simulink model "puma_pbvs"  (R2016a)
settings: Solver=ode45  StartTime=0.0  StopTime=20.0  RelTol=1e-3
InitFcn:
  | mdl_puma560
  | camera = CentralCamera('default');
  | P = mkgrid(2, 0.5, troty(pi/2)*transl(0,0,2.5));
  | q0 = [0 pi/4 pi 0 pi/4 -pi/4]';
undefined symbols (not defined in the file or in its folder): get_T_c_to_cdes
libraries: roblocks x8
settings Model: ExtModeTrigMode=oneshot  ExtModeArmWhenConnect=off  Creator=pic  LastModifiedBy=magiccjae
settings DataIOCC: SaveFormat=StructureWithTime  SignalLoggingSaveFormat=ModelDataLogs  ReturnWorkspaceOutputs=on
settings OptimizationCC: BlockReduction=off  BooleanDataType=off  ExpressionDepthLimit=2147483647  InitFltsAndDblsToZero=on
settings DebuggingCC: SaveWithParameterizedLinksMsg=none  UnderspecifiedInitializationDetection=Classic  MergeDetectMultiDrivingBlocksExec=none  SignalResolutionControl=TryResolveAllWithWarning  MultiTaskDSMMsg=warning  MultiTaskCondExecSysMsg=none  FcnCallInpInsideContextMsg=UseLocalSettings  StateNameClashWarn=warning
settings HardwareCC: ProdBitPerPointer=32  ProdLargestAtomicFloat=None  ProdIntDivRoundTo=Undefined  ProdEndianess=Unspecified  ProdWordSize=32  ProdHWDeviceType=32-bit Generic  TargetUnknown=on
settings ModelReferenceCC: PropagateSignalLabelsOutOfModel=off
settings GRTTargetCC: ModelReferenceCompliant=off  CompOptLevelCompliant=off  CombineOutputUpdateFcns=off  MatFileLogging=off  GRTInterface=on
settings ConfigComp: CovModelRefEnable=Off  CovSFcnEnable=off

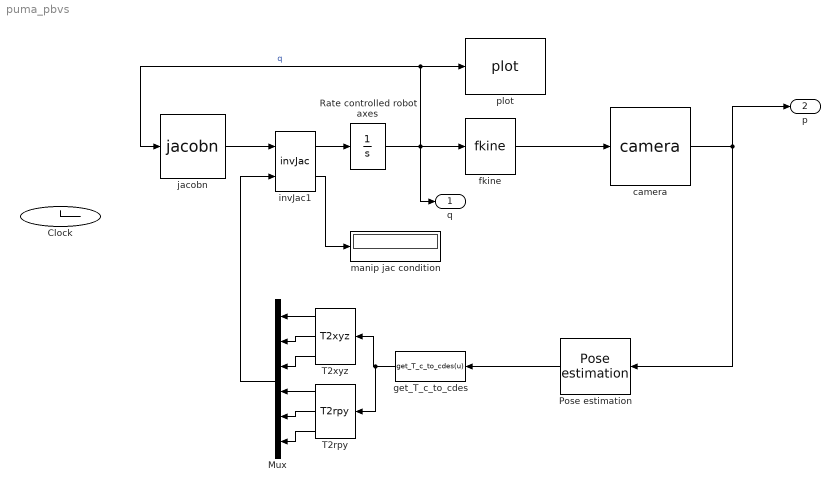
== system puma_pbvs ==
  Clock : Clock
  Mux : Mux  Inputs=6
  Pose estimation : roblocks/Vision/Pose estimation  cam=camera  P=P
  Rate controlled robot axes : Integrator  InitialCondition=q0
  T2rpy : roblocks/Transform Conversion/T2rpy
  T2xyz : roblocks/Transform Conversion/T2xyz
  camera : roblocks/Vision/camera  cam=camera  points=P
  fkine : roblocks/Kinematics/fkine  robot=p560
  get_T_c_to_cdes : MATLABFcn  MATLABFcn=get_T_c_to_cdes(u)  OutputDimensions=[4,4]  Output1D=off
  invJac1 : roblocks/Vision/invJac
  jacobn : roblocks/Kinematics/jacobn  robot=p560
  manip jac condition : Display
  plot : roblocks/Robot Graphics/plot  robot=p560  fps=25  holdplot=on
  q : Outport
  p : Outport  Port=2
  wires:
  Rate controlled robot axes/1 -> fkine/1, q/1, jacobn/1, plot/1  "q"
  jacobn/1 -> invJac1/1
  invJac1/1 -> Rate controlled robot axes/1
  fkine/1 -> camera/1
  camera/1 -> Pose estimation/1, p/1
  invJac1/2 -> manip jac condition/1
  Pose estimation/1 -> get_T_c_to_cdes/1
  get_T_c_to_cdes/1 -> T2rpy/1, T2xyz/1
  T2xyz/1 -> Mux/1
  T2xyz/2 -> Mux/2
  T2xyz/3 -> Mux/3
  T2rpy/1 -> Mux/4
  T2rpy/2 -> Mux/5
  T2rpy/3 -> Mux/6
  Mux/1 -> invJac1/2
